simulink model "question3(1)"  (R2016a)
settings: Solver=VariableStepAuto  StartTime=0.0  StopTime=0.1  RelTol=1e-3
libraries: powerlib x15, powerlib_meascontrol x6
settings Model: Creator=Think  LastModifiedBy=lll
settings DataIOCC: LimitDataPoints=on
settings DebuggingCC: AllowSymbolicDim=off
settings ModelReferenceCC: PropagateSignalLabelsOutOfModel=off
settings GRTTargetCC: GeneratePreprocessorConditionals=Use local settings

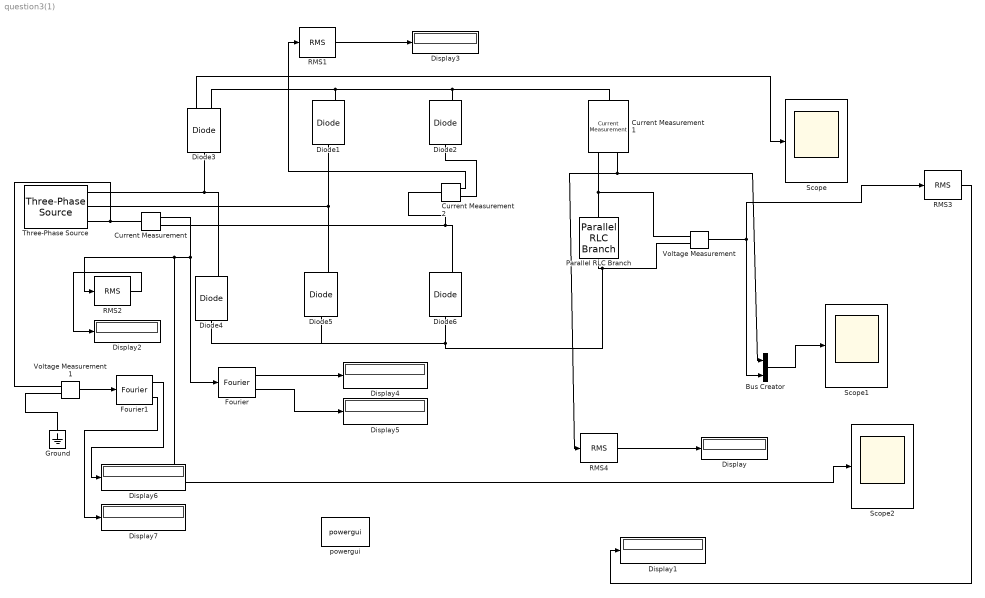
== system question3(1) ==
  Bus Creator : BusCreator  Inputs=2
  Current Measurement : powerlib/Measurements/Current Measurement  PhasorSimulation=off  OutputType=Complex  PSBequivalent=0
  Current Measurement1 : powerlib/Measurements/Current Measurement  PhasorSimulation=off  OutputType=Complex  PSBequivalent=0
  Current Measurement2 : powerlib/Measurements/Current Measurement  PhasorSimulation=off  OutputType=Complex  PSBequivalent=0
  Diode{1..6} (6 alike) : powerlib/Power Electronics/Diode  Ron=0.001  Lon=0  Vf=0.8  IC=0  UseSnubber=off  Rs=500  Cs=250e-9  Measurements=on
  Display{,1..7} (8 alike) : Display
  Fourier : powerlib_meascontrol/Measurements/Fourier  Freq=50  n=1  InInit=[0, 0]  Ts=0
  Fourier1 : powerlib_meascontrol/Measurements/Fourier  Freq=50  n=1  InInit=[0, 0]  Ts=0
  Ground : powerlib/Elements/Ground  LConnTagsString=a
  Parallel RLC Branch : powerlib/Elements/Parallel RLC Branch  LConnTagsString=a  RConnTagsString=__new0  BranchType=RC  Resistance=80  Inductance=9999999999999999999999999999999999999  SetiL0=off  InitialCurrent=0  Capacitance=0.0075  Setx0=off  InitialVoltage=0  Measurements=None
  RMS{1..4} (4 alike) : powerlib_meascontrol/Measurements/RMS  TrueRMS=on  Freq=50  RMSInit=120  Ts=0
  Scope : Scope
  Scope1 : Scope
  Scope2 : Scope
  Three-Phase Source : powerlib/Electrical Sources/Three-Phase Source  InternalConnection=Yg  VoltagePhases=off  Voltage=380  PhaseAngle=0  Voltage_phases=[25e3 25e3 25e3]/sqrt(3)  PhaseAngles_phases=[0 -120 +120]  Frequency=50  NonIdealSource=on  SpecifyImpedance=off  Resistance=0  Inductance=0  ShortCircuitLevel=100e6  BaseVoltage=25e3  XRratio=7  BusType=swing  Pref=10e3  Qref=0  Prefabc=[10e3, 10e3, 10e3]  Qrefabc=[0, 0, 0]  Qmin=-inf  Qmax=inf
  Voltage Measurement : powerlib/Measurements/Voltage Measurement  PhasorSimulation=off  OutputType=Complex  PSBequivalent=0
  Voltage Measurement1 : powerlib/Measurements/Voltage Measurement  PhasorSimulation=off  OutputType=Complex  PSBequivalent=0
  powergui : powerlib/powergui  Priority=1  SimulationMode=Continuous  SolverType=Tustin/Backward Euler (TBE)  SampleTime=50e-6  frequency=60  SPID=off  DisableSnubberDevices=off  DisableRonSwitches=off  DisableVfSwitches=off  SwTol=0  DisplayEquations=off  Interpol=off  ExternalGateDelay=off  methode=off  Ts=10  FunctionMessages=off  echomessages=off  HookPort=off  EnableUseOfTLC=off  x0status=blocks  frequencyindice=50  Pbase=100e6  ErrMax=1e-4  Iterations=50  UnitsV=V  UnitsW=MW  buscounter=0  RestoreLinks=warning  ResistiveCurrentMeasurement=off  Frange=[0:2:500]  Ylog=off  Xlog=on  ShowGrid=off  save=off  variable=ZData  structure=Data2  ZoomFFT=off  StartTime=0.06  cycles=1  DisplayStyle=1  fundamental=50  FreqAxis=off  MaxFrequency=1000  frequencyindicesteady=1  RmsSteady=1  display=off
  wires:
  RMS3/1 -> Display1/1
  RMS4/1 -> Display/1
  Current Measurement/1 -> Fourier/1, Scope2/1, RMS2/1
  RMS2/1 -> Display2/1
  Current Measurement2/1 -> RMS1/1
  RMS1/1 -> Display3/1
  Voltage Measurement/1 -> RMS3/1, Bus Creator/2
  Diode3/1 -> Scope/1
  Bus Creator/1 -> Scope1/1
  Current Measurement1/1 -> RMS4/1, Bus Creator/1
  Fourier/1 -> Display4/1
  Fourier/2 -> Display5/1
  Fourier1/1 -> Display6/1
  Fourier1/2 -> Display7/1
  Voltage Measurement1/1 -> Fourier1/1
  connections:
  Three-Phase Source/RConn1 -- Diode4/RConn1 -- Diode3/LConn1
  Three-Phase Source/RConn2 -- Diode5/RConn1 -- Diode1/LConn1
  Current Measurement/RConn1 -- Diode6/RConn1 -- Current Measurement2/LConn1
  Current Measurement1/RConn1 -- Voltage Measurement/LConn1 -- Parallel RLC Branch/RConn1
  Current Measurement/LConn1 -- Voltage Measurement1/LConn1 -- Three-Phase Source/RConn3
  Current Measurement1/LConn1 -- Diode3/RConn1 -- Diode1/RConn1 -- Diode2/RConn1
  Diode2/LConn1 -- Current Measurement2/RConn1
  Voltage Measurement/LConn2 -- Diode6/LConn1 -- Diode5/LConn1 -- Diode4/LConn1 -- Parallel RLC Branch/LConn1
  Ground/LConn1 -- Voltage Measurement1/LConn2
